simulink model "DC_motor"  (R2021a)
settings: Solver=VariableStepAuto  StartTime=0.0  StopTime=1  RelTol=1e-3
libraries: fl_lib x45, nesl_utility x21, ee_lib x15
settings Model: Creator=vomi  LastModifiedBy=vomi

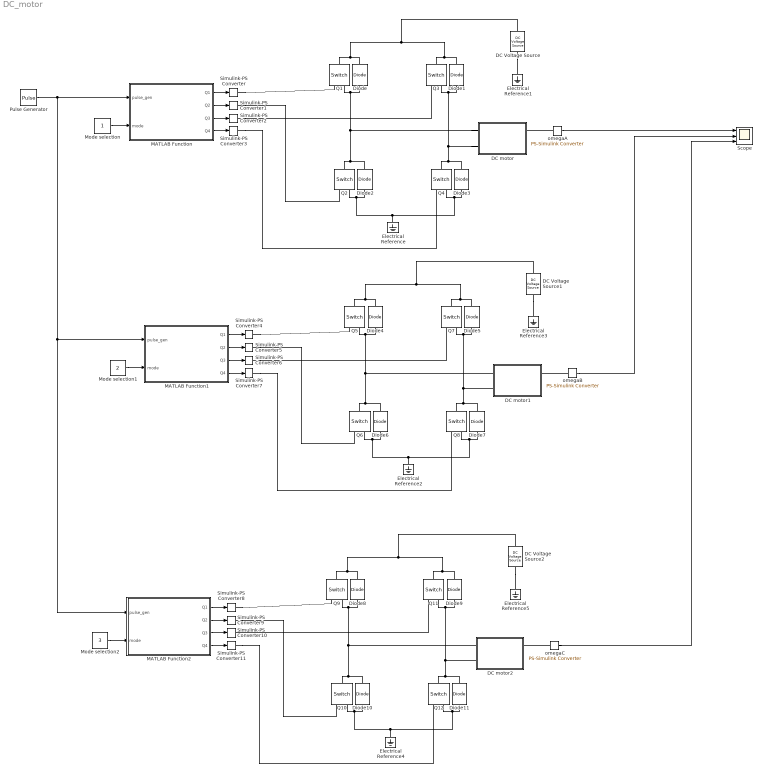
== system DC_motor ==
  DC Voltage Source : ee_lib/Additional Components/SPICE Sources/DC Voltage Source  DC=14.4 V
  DC Voltage Source1 : ee_lib/Additional Components/SPICE Sources/DC Voltage Source  DC=14.4 V
  DC Voltage Source2 : ee_lib/Additional Components/SPICE Sources/DC Voltage Source  DC=14.4 V
  DC motor : Subsystem
  DC motor1 : Subsystem
  DC motor2 : Subsystem
  Diode{,1..11} (12 alike) : ee_lib/Semiconductors & Converters/Diode  ModelType=ee.enum.diode.modelType.pwl  IfMat=[.07, .12, .19, 1.75, 4.24, 7.32, 11.2; .16, .3, .72, 2.14, 4.02, 6.35, 9.12] A  TjVec=[25, 125] degC  VfVec=[.5, .7, .9, 1.3, 1.7, 2.1, 2.5] V  Vf=0.6 V  Ron=0.3 Ohm  Goff=1e-8 S  prmExp=ee.enum.diode.expParam.useTwo  I12=[.0137, .545] A  V12=[.6, .7] V  IS=1e-12 A  ec=1  I1=0.0137 A  V1=0.6 V  RS=0 Ohm  Tmeas=25 degC  N_series=1  N_parallel=1  Rz=0.3 Ohm  BV=inf V  C_param=ee.enum.diode.capParam.fixed  CJ=5 pF  CJ0=5 pF  VJ=1 V  Mgrad=0.5  Vvec=[.1, 10, 100] V  Cvec=[3.5, 1, .4] pF  FC=0.5  Q_param=ee.enum.diode.recoveryParam.off  iRM=-7.15 A  iF=4 A  didt=-750 A/us  trr_factor=3  trr=115 ns  Qrr=150 s*nA  TT=50 ns  tau=100 ns  T_param=ee.enum.diode.temperatureParam.off  IS_T2=1.25e-7 A  I1_T2=0.245 A  V1_T2=0.5 V  Tmeas2=125 degC  EG_param=ee.enum.diode.egapParam.material_si  EG=1.11 eV  XTI_param=ee.enum.diode.xtiParam.pn  XTI=3  dBVdT=0 V/K  enable_faults=ee.enum.faults.faultEnable.no  fault_action=ee.enum.faults.faultAction.none  fault_types=ee.enum.diode.faults.open  tau_fault=1e-3 s  IfMat_faulted=[.07, .12, .19, 1.75, 4.24, 7.32, 11.2; .16, .3, .72, 2.14, 4.02, 6.35, 9.12] A  VfVec_faulted=[.5, .7, .9, 1.3, 1.7, 2.1, 2.5] V  Ropen_faulted=1000 Ohm  Gshort_faulted=1000 1/Ohm  Vf_faulted=0.6 V  Ron_faulted=0.3 Ohm  Goff_faulted=1e-8 S  I12_faulted=[.0137, .545] A  V12_faulted=[.6, .7] V  IS_faulted=1e-12 A  ec_faulted=1  I1_faulted=0.0137 A  V1_faulted=0.6 V  RS_faulted=0 Ohm  Rz_faulted=0.3 Ohm  BV_faulted=inf V  Cscale_faulted=100  enable_temporal_fault=ee.enum.faults.faultEnable.no  t_fault=inf s  enable_behavioral_fault=ee.enum.faults.faultEnable.no  max_permissible_voltage=inf V  n_fail_on_voltage=1  max_permissible_current=inf A  t_fail_on_current=1 s  max_permissible_dVdt=inf V/s  Tdevice=25 degC  i_specify=off  i_priority=None  i=0 A  i_nominal_specify=off  i_nominal_unit=A  i_nominal_value=1  v_specify=off  v_priority=None  v=0 V  v_nominal_specify=off  v_nominal_unit=V  v_nominal_value=1  i_diode_specify=off  i_diode_priority=None  i_diode=0 A  i_diode_nominal_specify=off  i_diode_nominal_unit=A  i_diode_nominal_value=1  v_diode_specify=off  v_diode_priority=None  v_diode=0 V  v_diode_nominal_specify=off  v_diode_nominal_unit=V  v_diode_nominal_value=1  i_capacitor_specify=off  i_capacitor_priority=None  i_capacitor=0 A  i_capacitor_nominal_specify=off  i_capacitor_nominal_unit=A  i_capacitor_nominal_value=1  v_capacitor_specify=off  v_capacitor_priority=None  v_capacitor=0 V  v_capacitor_nominal_specify=off  v_capacitor_nominal_unit=V  v_capacitor_nominal_value=1  power_dissipated_specify=off  power_dissipated_priority=None  power_dissipated=0 W  power_dissipated_nominal_specify=off  power_dissipated_nominal_unit=W  power_dissipated_nominal_value=1  max_permissible_temperature=inf K  t_fail_on_temperature=1 s  thermal_network_parameterization=ee.enum.thermalNetworkTopology.cauer  Rth=[0, 10] K/W  Rth_Foster=[4, 6] K/W  thermal_mass_parameterization=ee.enum.thermalNetwork.timeconstant  thermal_mass=[0, 1] J/K  thermal_mass_Foster=[1.5, 3] J/K  thermal_time_constant=[0, 10] s  thermal_time_constant_Foster=[6, 18] s  thermal_mass_initial_temperatures=[25, 25] degC
  Electrical Reference{,1..5} (6 alike) : fl_lib/Electrical/Electrical Elements/Electrical Reference
  MATLAB Function : MATLAB Function  TreatAsAtomicUnit=on
  MATLAB Function1 : MATLAB Function  TreatAsAtomicUnit=on
  MATLAB Function2 : MATLAB Function  TreatAsAtomicUnit=on
  Mode selection : Constant
  Mode selection1 : Constant  Value=2
  Mode selection2 : Constant  Value=3
  Pulse Generator : DiscretePulseGenerator  PulseType=Time based  Period=1/25.3e3  PulseWidth=30
  Q{1..12} (12 alike) : fl_lib/Electrical/Electrical Elements/Switch  R_closed=0.01 Ohm  G_open=1e-8 1/Ohm  Threshold=0.5  i_specify=off  i_priority=None  i=0 A  i_nominal_specify=off  i_nominal_unit=A  i_nominal_value=1  v_specify=off  v_priority=None  v=0 V  v_nominal_specify=off  v_nominal_unit=V  v_nominal_value=1
  Scope : Scope  NumInputPorts=3
  Simulink-PS Converter{,1..11} (12 alike) : nesl_utility/Simulink-PS Converter  PhysicalDomain=network_engine_domain  SubClassName=ps_input  LeftPortType=input  RightPortType=output  PseudoPeriodic=off  Frequencies=[]  NoiseDistribution=none  NoiseParameters=[]  Unit=1  AffineConversion=off  FilteringAndDerivatives=provide  SimscapeFilterOrder=1  InputFilterTimeConstant=0.001  UdotUserProvided=0
      settings: SourceProductBaseCode=PW,SS
  omegaA : nesl_utility/PS-Simulink Converter  PhysicalDomain=network_engine_domain  SubClassName=ps_output  LeftPortType=input  RightPortType=output  PseudoPeriodic=off  Frequencies=[]  Unit=inherit  AffineConversion=off
      settings: SourceProductBaseCode=PW,SS
  omegaB : nesl_utility/PS-Simulink Converter  PhysicalDomain=network_engine_domain  SubClassName=ps_output  LeftPortType=input  RightPortType=output  PseudoPeriodic=off  Frequencies=[]  Unit=inherit  AffineConversion=off
      settings: SourceProductBaseCode=PW,SS
  omegaC : nesl_utility/PS-Simulink Converter  PhysicalDomain=network_engine_domain  SubClassName=ps_output  LeftPortType=input  RightPortType=output  PseudoPeriodic=off  Frequencies=[]  Unit=inherit  AffineConversion=off
      settings: SourceProductBaseCode=PW,SS
  wires:
  omegaA/1 -> Scope/1
  MATLAB Function/2(Q2) -> Simulink-PS Converter1/1
  MATLAB Function/4(Q4) -> Simulink-PS Converter3/1
  MATLAB Function/3(Q3) -> Simulink-PS Converter2/1
  MATLAB Function/1(Q1) -> Simulink-PS Converter/1
  Mode selection/1 -> MATLAB Function/2(mode)
  MATLAB Function1/4(Q4) -> Simulink-PS Converter7/1
  MATLAB Function1/1(Q1) -> Simulink-PS Converter4/1
  MATLAB Function1/2(Q2) -> Simulink-PS Converter5/1
  Mode selection1/1 -> MATLAB Function1/2(mode)
  MATLAB Function1/3(Q3) -> Simulink-PS Converter6/1
  omegaB/1 -> Scope/2
  Pulse Generator/1 -> MATLAB Function1/1(pulse_gen), MATLAB Function2/1(pulse_gen), MATLAB Function/1(pulse_gen)
  Mode selection2/1 -> MATLAB Function2/2(mode)
  MATLAB Function2/1(Q1) -> Simulink-PS Converter8/1
  MATLAB Function2/4(Q4) -> Simulink-PS Converter11/1
  omegaC/1 -> Scope/3
  MATLAB Function2/3(Q3) -> Simulink-PS Converter10/1
  MATLAB Function2/2(Q2) -> Simulink-PS Converter9/1
  connections:
  omegaA/LConn1 -- DC motor/RConn1
  Diode2/RConn1 -- DC motor/LConn1 -- Diode/LConn1 -- Q1/RConn2 -- Q2/LConn1
  Diode/RConn1 -- Q1/LConn1 -- Q3/LConn1 -- Diode1/RConn1 -- DC Voltage Source/LConn1
  Diode3/RConn1 -- DC motor/LConn2 -- Diode1/LConn1 -- Q3/RConn2 -- Q4/LConn1
  Q2/RConn2 -- Electrical Reference/LConn1 -- Diode3/LConn1 -- Q4/RConn2 -- Diode2/LConn1
  DC Voltage Source/RConn1 -- Electrical Reference1/LConn1
  Simulink-PS Converter/RConn1 -- Q1/RConn1
  Simulink-PS Converter1/RConn1 -- Q2/RConn1
  Simulink-PS Converter2/RConn1 -- Q3/RConn1
  Simulink-PS Converter3/RConn1 -- Q4/RConn1
  DC Voltage Source1/LConn1 -- Q7/LConn1 -- Diode5/RConn1 -- Diode4/RConn1 -- Q5/LConn1
  Q7/RConn2 -- Diode7/RConn1 -- Q8/LConn1 -- DC motor1/LConn2 -- Diode5/LConn1
  Q8/RConn2 -- Diode6/LConn1 -- Q6/RConn2 -- Electrical Reference2/LConn1 -- Diode7/LConn1
  Q5/RConn2 -- Diode6/RConn1 -- Q6/LConn1 -- DC motor1/LConn1 -- Diode4/LConn1
  Simulink-PS Converter6/RConn1 -- Q7/RConn1
  omegaB/LConn1 -- DC motor1/RConn1
  Simulink-PS Converter5/RConn1 -- Q6/RConn1
  DC Voltage Source1/RConn1 -- Electrical Reference3/LConn1
  Simulink-PS Converter4/RConn1 -- Q5/RConn1
  Simulink-PS Converter7/RConn1 -- Q8/RConn1
  Q9/RConn2 -- Diode10/RConn1 -- Q10/LConn1 -- DC motor2/LConn1 -- Diode8/LConn1
  Q12/RConn2 -- Diode11/LConn1 -- Electrical Reference4/LConn1 -- Diode10/LConn1 -- Q10/RConn2
  Q11/RConn2 -- Diode9/LConn1 -- Diode11/RConn1 -- Q12/LConn1 -- DC motor2/LConn2
  Q9/LConn1 -- Diode8/RConn1 -- DC Voltage Source2/LConn1 -- Q11/LConn1 -- Diode9/RConn1
  Simulink-PS Converter9/RConn1 -- Q10/RConn1
  Simulink-PS Converter8/RConn1 -- Q9/RConn1
  Simulink-PS Converter10/RConn1 -- Q11/RConn1
  DC Voltage Source2/RConn1 -- Electrical Reference5/LConn1
  omegaC/LConn1 -- DC motor2/RConn1
  Simulink-PS Converter11/RConn1 -- Q12/RConn1

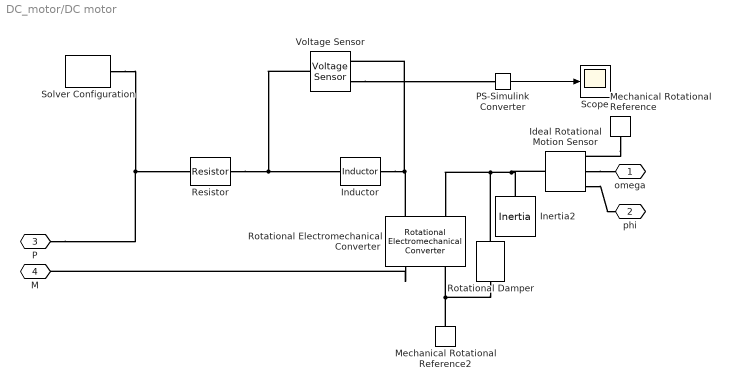
== system DC_motor/DC motor ==
  Ideal Rotational Motion Sensor : fl_lib/Mechanical/Mechanical Sensors/Ideal Rotational Motion Sensor  wrap_angle=simscape.enum.onoff.off  offset=0 rad
  Inductor : fl_lib/Electrical/Electrical Elements/Inductor  l=0.4 mH  r=0 Ohm  g=1e-9 1/Ohm  i_specify=off  i_priority=None  i=0 A  i_nominal_specify=off  i_nominal_unit=A  i_nominal_value=1  v_specify=off  v_priority=None  v=0 V  v_nominal_specify=off  v_nominal_unit=V  v_nominal_value=1  i_L_specify=off  i_L_priority=High  i_L=0 A  i_L_nominal_specify=off  i_L_nominal_unit=A  i_L_nominal_value=1
  Inertia2 : fl_lib/Mechanical/Rotational Elements/Inertia  inertia=71.4e-7 kg*m^2  num_ports=foundation.enum.numPorts2.one  w_specify=off  w_priority=High  w=0 rad/s  w_nominal_specify=off  w_nominal_unit=rad/s  w_nominal_value=1  t_specify=off  t_priority=None  t=0 N*m  t_nominal_specify=off  t_nominal_unit=N*m  t_nominal_value=1
  Mechanical Rotational Reference : fl_lib/Mechanical/Rotational Elements/Mechanical Rotational Reference
  Mechanical Rotational Reference2 : fl_lib/Mechanical/Rotational Elements/Mechanical Rotational Reference
  PS-Simulink Converter : nesl_utility/PS-Simulink Converter  PhysicalDomain=network_engine_domain  SubClassName=ps_output  LeftPortType=input  RightPortType=output  PseudoPeriodic=off  Frequencies=[]  Unit=inherit  AffineConversion=off
      settings: SourceProductBaseCode=PW,SS
  Resistor : fl_lib/Electrical/Electrical Elements/Resistor  R=2.20 Ohm  i_specify=off  i_priority=None  i=0 A  i_nominal_specify=off  i_nominal_unit=A  i_nominal_value=1  v_specify=off  v_priority=None  v=0 V  v_nominal_specify=off  v_nominal_unit=V  v_nominal_value=1
  Rotational Electromechanical Converter : fl_lib/Electrical/Electrical Elements/Rotational Electromechanical Converter  K=5.40e-3 V/rpm  i_specify=off  i_priority=None  i=0 A  i_nominal_specify=off  i_nominal_unit=A  i_nominal_value=1  v_specify=off  v_priority=None  v=0 V  v_nominal_specify=off  v_nominal_unit=V  v_nominal_value=1  t_specify=off  t_priority=None  t=0 N*m  t_nominal_specify=off  t_nominal_unit=N*m  t_nominal_value=1  w_specify=off  w_priority=None  w=0 rad/s  w_nominal_specify=off  w_nominal_unit=rad/s  w_nominal_value=1
  Rotational Damper : fl_lib/Mechanical/Rotational Elements/Rotational Damper  D=0.00002 N*m/(rad/s)  w_specify=off  w_priority=None  w=0 rad/s  w_nominal_specify=off  w_nominal_unit=rad/s  w_nominal_value=1  t_specify=off  t_priority=None  t=0 N*m  t_nominal_specify=off  t_nominal_unit=N*m  t_nominal_value=1
  Scope : Scope
  Solver Configuration : nesl_utility/Solver Configuration  PhysicalDomain=network_engine_domain  SubClassName=solver  LeftPortType=input  RightPortType=generic  Tones=[]  Harmonics=[]  SimulateNoise=off  Profile=off  UseLocalSampling=off  EnableSwitchedLinearOptims=on  FrequencyDomain=off  UseCCode=off  RelTol=0.001  AbsTol=1e-06  MinStep=1e-09  ToWorkspace=off  RevertToSquareIcSolve=off  NumHomotopyIterations=100  PhasorMode=off  PhasorModeNumHarmonics=1  DoDC=off  ResidualTolerance=1e-09  UseLocalSolver=off  LocalSolverChoice=NE_BACKWARD_EULER_ADVANCER  LocalSolverSampleTime=0.001  DoFixedCost=off  MaxNonlinIter=3  MaxModeIter=2  ComputeImpulses=off  ImpulseIterations=2  LinearAlgebra=auto  EquationFormulation=NE_TIME_EF  DelaysMemoryBudget=1024  AutomaticFiltering=on  FilteringTimeConstant=0.001  PartitionStorageMethod=AS_NEEDED  PartitionMemoryBudget=1024  PartitionMethod=ROBUST
      settings: SourceProductBaseCode=PW,SS
  Voltage Sensor : fl_lib/Electrical/Electrical Sensors/Voltage Sensor
  omega : PMIOPort  Side=Right
  phi : PMIOPort  Port=2  Side=Right
  P : PMIOPort  Port=3  Side=Left
  M : PMIOPort  Port=4  Side=Left
  wires:
  PS-Simulink Converter/1 -> Scope/1
  connections:
  Inductor/RConn1 -- Rotational Electromechanical Converter/LConn1 -- Voltage Sensor/RConn2
  Ideal Rotational Motion Sensor/RConn2 -- omega/RConn1
  Resistor/RConn1 -- Voltage Sensor/LConn1 -- Inductor/LConn1
  Inertia2/LConn1 -- Ideal Rotational Motion Sensor/LConn1 -- Rotational Damper/RConn1 -- Rotational Electromechanical Converter/LConn2
  Rotational Electromechanical Converter/RConn1 -- M/RConn1
  Voltage Sensor/RConn1 -- PS-Simulink Converter/LConn1
  Mechanical Rotational Reference/LConn1 -- Ideal Rotational Motion Sensor/RConn1
  Solver Configuration/RConn1 -- P/RConn1 -- Resistor/LConn1
  Mechanical Rotational Reference2/LConn1 -- Rotational Damper/LConn1 -- Rotational Electromechanical Converter/RConn2
  Ideal Rotational Motion Sensor/RConn3 -- phi/RConn1

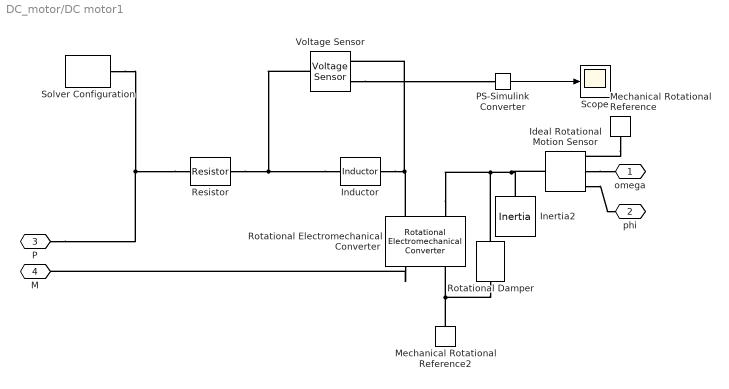
== system DC_motor/DC motor1 ==
  Ideal Rotational Motion Sensor : fl_lib/Mechanical/Mechanical Sensors/Ideal Rotational Motion Sensor  wrap_angle=simscape.enum.onoff.off  offset=0 rad
  Inductor : fl_lib/Electrical/Electrical Elements/Inductor  l=0.4 mH  r=0 Ohm  g=1e-9 1/Ohm  i_specify=off  i_priority=None  i=0 A  i_nominal_specify=off  i_nominal_unit=A  i_nominal_value=1  v_specify=off  v_priority=None  v=0 V  v_nominal_specify=off  v_nominal_unit=V  v_nominal_value=1  i_L_specify=off  i_L_priority=High  i_L=0 A  i_L_nominal_specify=off  i_L_nominal_unit=A  i_L_nominal_value=1
  Inertia2 : fl_lib/Mechanical/Rotational Elements/Inertia  inertia=71.4e-7 kg*m^2  num_ports=foundation.enum.numPorts2.one  w_specify=off  w_priority=High  w=0 rad/s  w_nominal_specify=off  w_nominal_unit=rad/s  w_nominal_value=1  t_specify=off  t_priority=None  t=0 N*m  t_nominal_specify=off  t_nominal_unit=N*m  t_nominal_value=1
  Mechanical Rotational Reference : fl_lib/Mechanical/Rotational Elements/Mechanical Rotational Reference
  Mechanical Rotational Reference2 : fl_lib/Mechanical/Rotational Elements/Mechanical Rotational Reference
  PS-Simulink Converter : nesl_utility/PS-Simulink Converter  PhysicalDomain=network_engine_domain  SubClassName=ps_output  LeftPortType=input  RightPortType=output  PseudoPeriodic=off  Frequencies=[]  Unit=inherit  AffineConversion=off
      settings: SourceProductBaseCode=PW,SS
  Resistor : fl_lib/Electrical/Electrical Elements/Resistor  R=2.20 Ohm  i_specify=off  i_priority=None  i=0 A  i_nominal_specify=off  i_nominal_unit=A  i_nominal_value=1  v_specify=off  v_priority=None  v=0 V  v_nominal_specify=off  v_nominal_unit=V  v_nominal_value=1
  Rotational Electromechanical Converter : fl_lib/Electrical/Electrical Elements/Rotational Electromechanical Converter  K=5.40e-3 V/rpm  i_specify=off  i_priority=None  i=0 A  i_nominal_specify=off  i_nominal_unit=A  i_nominal_value=1  v_specify=off  v_priority=None  v=0 V  v_nominal_specify=off  v_nominal_unit=V  v_nominal_value=1  t_specify=off  t_priority=None  t=0 N*m  t_nominal_specify=off  t_nominal_unit=N*m  t_nominal_value=1  w_specify=off  w_priority=None  w=0 rad/s  w_nominal_specify=off  w_nominal_unit=rad/s  w_nominal_value=1
  Rotational Damper : fl_lib/Mechanical/Rotational Elements/Rotational Damper  D=0.00002 N*m/(rad/s)  w_specify=off  w_priority=None  w=0 rad/s  w_nominal_specify=off  w_nominal_unit=rad/s  w_nominal_value=1  t_specify=off  t_priority=None  t=0 N*m  t_nominal_specify=off  t_nominal_unit=N*m  t_nominal_value=1
  Scope : Scope
  Solver Configuration : nesl_utility/Solver Configuration  PhysicalDomain=network_engine_domain  SubClassName=solver  LeftPortType=input  RightPortType=generic  Tones=[]  Harmonics=[]  SimulateNoise=off  Profile=off  UseLocalSampling=off  EnableSwitchedLinearOptims=on  FrequencyDomain=off  UseCCode=off  RelTol=0.001  AbsTol=1e-06  MinStep=1e-09  ToWorkspace=off  RevertToSquareIcSolve=off  NumHomotopyIterations=100  PhasorMode=off  PhasorModeNumHarmonics=1  DoDC=off  ResidualTolerance=1e-09  UseLocalSolver=off  LocalSolverChoice=NE_BACKWARD_EULER_ADVANCER  LocalSolverSampleTime=0.001  DoFixedCost=off  MaxNonlinIter=3  MaxModeIter=2  ComputeImpulses=off  ImpulseIterations=2  LinearAlgebra=auto  EquationFormulation=NE_TIME_EF  DelaysMemoryBudget=1024  AutomaticFiltering=on  FilteringTimeConstant=0.001  PartitionStorageMethod=AS_NEEDED  PartitionMemoryBudget=1024  PartitionMethod=ROBUST
      settings: SourceProductBaseCode=PW,SS
  Voltage Sensor : fl_lib/Electrical/Electrical Sensors/Voltage Sensor
  omega : PMIOPort  Side=Right
  phi : PMIOPort  Port=2  Side=Right
  P : PMIOPort  Port=3  Side=Left
  M : PMIOPort  Port=4  Side=Left
  wires:
  PS-Simulink Converter/1 -> Scope/1
  connections:
  Inductor/RConn1 -- Voltage Sensor/RConn2 -- Rotational Electromechanical Converter/LConn1
  Ideal Rotational Motion Sensor/RConn2 -- omega/RConn1
  Inductor/LConn1 -- Resistor/RConn1 -- Voltage Sensor/LConn1
  Rotational Electromechanical Converter/LConn2 -- Ideal Rotational Motion Sensor/LConn1 -- Inertia2/LConn1 -- Rotational Damper/RConn1
  Rotational Electromechanical Converter/RConn1 -- M/RConn1
  Voltage Sensor/RConn1 -- PS-Simulink Converter/LConn1
  Mechanical Rotational Reference/LConn1 -- Ideal Rotational Motion Sensor/RConn1
  Resistor/LConn1 -- Solver Configuration/RConn1 -- P/RConn1
  Rotational Electromechanical Converter/RConn2 -- Mechanical Rotational Reference2/LConn1 -- Rotational Damper/LConn1
  Ideal Rotational Motion Sensor/RConn3 -- phi/RConn1

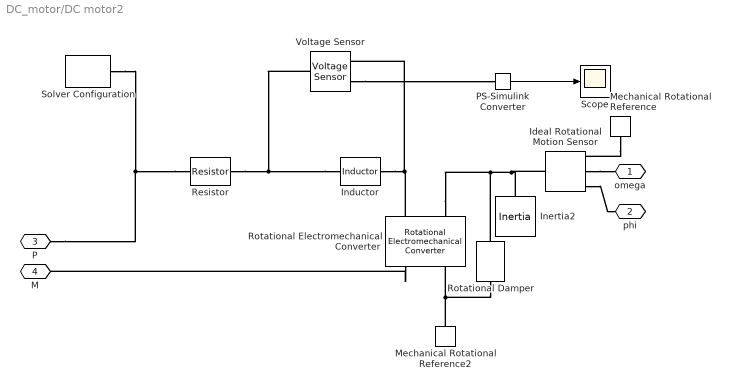
== system DC_motor/DC motor2 ==
  Ideal Rotational Motion Sensor : fl_lib/Mechanical/Mechanical Sensors/Ideal Rotational Motion Sensor  wrap_angle=simscape.enum.onoff.off  offset=0 rad
  Inductor : fl_lib/Electrical/Electrical Elements/Inductor  l=0.4 mH  r=0 Ohm  g=1e-9 1/Ohm  i_specify=off  i_priority=None  i=0 A  i_nominal_specify=off  i_nominal_unit=A  i_nominal_value=1  v_specify=off  v_priority=None  v=0 V  v_nominal_specify=off  v_nominal_unit=V  v_nominal_value=1  i_L_specify=off  i_L_priority=High  i_L=0 A  i_L_nominal_specify=off  i_L_nominal_unit=A  i_L_nominal_value=1
  Inertia2 : fl_lib/Mechanical/Rotational Elements/Inertia  inertia=71.4e-7 kg*m^2  num_ports=foundation.enum.numPorts2.one  w_specify=off  w_priority=High  w=0 rad/s  w_nominal_specify=off  w_nominal_unit=rad/s  w_nominal_value=1  t_specify=off  t_priority=None  t=0 N*m  t_nominal_specify=off  t_nominal_unit=N*m  t_nominal_value=1
  Mechanical Rotational Reference : fl_lib/Mechanical/Rotational Elements/Mechanical Rotational Reference
  Mechanical Rotational Reference2 : fl_lib/Mechanical/Rotational Elements/Mechanical Rotational Reference
  PS-Simulink Converter : nesl_utility/PS-Simulink Converter  PhysicalDomain=network_engine_domain  SubClassName=ps_output  LeftPortType=input  RightPortType=output  PseudoPeriodic=off  Frequencies=[]  Unit=inherit  AffineConversion=off
      settings: SourceProductBaseCode=PW,SS
  Resistor : fl_lib/Electrical/Electrical Elements/Resistor  R=2.20 Ohm  i_specify=off  i_priority=None  i=0 A  i_nominal_specify=off  i_nominal_unit=A  i_nominal_value=1  v_specify=off  v_priority=None  v=0 V  v_nominal_specify=off  v_nominal_unit=V  v_nominal_value=1
  Rotational Electromechanical Converter : fl_lib/Electrical/Electrical Elements/Rotational Electromechanical Converter  K=5.40e-3 V/rpm  i_specify=off  i_priority=None  i=0 A  i_nominal_specify=off  i_nominal_unit=A  i_nominal_value=1  v_specify=off  v_priority=None  v=0 V  v_nominal_specify=off  v_nominal_unit=V  v_nominal_value=1  t_specify=off  t_priority=None  t=0 N*m  t_nominal_specify=off  t_nominal_unit=N*m  t_nominal_value=1  w_specify=off  w_priority=None  w=0 rad/s  w_nominal_specify=off  w_nominal_unit=rad/s  w_nominal_value=1
  Rotational Damper : fl_lib/Mechanical/Rotational Elements/Rotational Damper  D=0.00002 N*m/(rad/s)  w_specify=off  w_priority=None  w=0 rad/s  w_nominal_specify=off  w_nominal_unit=rad/s  w_nominal_value=1  t_specify=off  t_priority=None  t=0 N*m  t_nominal_specify=off  t_nominal_unit=N*m  t_nominal_value=1
  Scope : Scope
  Solver Configuration : nesl_utility/Solver Configuration  PhysicalDomain=network_engine_domain  SubClassName=solver  LeftPortType=input  RightPortType=generic  Tones=[]  Harmonics=[]  SimulateNoise=off  Profile=off  UseLocalSampling=off  EnableSwitchedLinearOptims=on  FrequencyDomain=off  UseCCode=off  RelTol=0.001  AbsTol=1e-06  MinStep=1e-09  ToWorkspace=off  RevertToSquareIcSolve=off  NumHomotopyIterations=100  PhasorMode=off  PhasorModeNumHarmonics=1  DoDC=off  ResidualTolerance=1e-09  UseLocalSolver=off  LocalSolverChoice=NE_BACKWARD_EULER_ADVANCER  LocalSolverSampleTime=0.001  DoFixedCost=off  MaxNonlinIter=3  MaxModeIter=2  ComputeImpulses=off  ImpulseIterations=2  LinearAlgebra=auto  EquationFormulation=NE_TIME_EF  DelaysMemoryBudget=1024  AutomaticFiltering=on  FilteringTimeConstant=0.001  PartitionStorageMethod=AS_NEEDED  PartitionMemoryBudget=1024  PartitionMethod=ROBUST
      settings: SourceProductBaseCode=PW,SS
  Voltage Sensor : fl_lib/Electrical/Electrical Sensors/Voltage Sensor
  omega : PMIOPort  Side=Right
  phi : PMIOPort  Port=2  Side=Right
  P : PMIOPort  Port=3  Side=Left
  M : PMIOPort  Port=4  Side=Left
  wires:
  PS-Simulink Converter/1 -> Scope/1
  connections:
  Inductor/RConn1 -- Voltage Sensor/RConn2 -- Rotational Electromechanical Converter/LConn1
  Ideal Rotational Motion Sensor/RConn2 -- omega/RConn1
  Inductor/LConn1 -- Resistor/RConn1 -- Voltage Sensor/LConn1
  Rotational Electromechanical Converter/LConn2 -- Ideal Rotational Motion Sensor/LConn1 -- Inertia2/LConn1 -- Rotational Damper/RConn1
  Rotational Electromechanical Converter/RConn1 -- M/RConn1
  Voltage Sensor/RConn1 -- PS-Simulink Converter/LConn1
  Mechanical Rotational Reference/LConn1 -- Ideal Rotational Motion Sensor/RConn1
  Resistor/LConn1 -- Solver Configuration/RConn1 -- P/RConn1
  Rotational Electromechanical Converter/RConn2 -- Mechanical Rotational Reference2/LConn1 -- Rotational Damper/LConn1
  Ideal Rotational Motion Sensor/RConn3 -- phi/RConn1

== matlab function DC_motor/MATLAB Function1 ==
  data: pulse_gen input; Q1 output; mode input; Q2 output; Q3 output; Q4 output
function [Q1, Q2, Q3, Q4] = mosfet_drive(pulse_gen, mode)
if pulse_gen == 1 % spínáme
    drive = [1 0 0 1];
else % interval mezi sepnutími, brzdí se
    if mode == 1 % Mode A, Sign-Manitude
        drive = [1 0 1 0];    
    elseif mode == 2 % Mode B, Asynchronous Sign-magnitude
        drive = [1 0 0 0];
    else %Mode C, Lock Anti-Phase
        drive = [0 1 1 0];
    end
end
Q1 = drive(1);
Q2 = drive(2);
Q3 = drive(3);
Q4 = drive(4);
end

== matlab function DC_motor/MATLAB Function ==
  data: pulse_gen input; Q1 output; mode input; Q2 output; Q3 output; Q4 output
function [Q1, Q2, Q3, Q4] = mosfet_drive(pulse_gen, mode)
if pulse_gen == 1 % spínáme
    drive = [1 0 0 1];
else % interval mezi sepnutími, brzdí se
    if mode == 1 % Mode A, Sign-Manitude
        drive = [1 0 1 0];    
    elseif mode == 2 % Mode B, Asynchronous Sign-magnitude
        drive = [1 0 0 0];
    else %Mode C, Lock Anti-Phase
        drive = [0 1 1 0];
    end
end
Q1 = drive(1);
Q2 = drive(2);
Q3 = drive(3);
Q4 = drive(4);
end

== matlab function DC_motor/MATLAB Function2 ==
  data: pulse_gen input; Q1 output; mode input; Q2 output; Q3 output; Q4 output
function [Q1, Q2, Q3, Q4] = mosfet_drive(pulse_gen, mode)
if pulse_gen == 1 % spínáme
    drive = [1 0 0 1];
else % interval mezi sepnutími, brzdí se
    if mode == 1 % Mode A, Sign-Manitude
        drive = [1 0 1 0];    
    elseif mode == 2 % Mode B, Asynchronous Sign-magnitude
        drive = [1 0 0 0];
    else %Mode C, Lock Anti-Phase
        drive = [0 1 1 0];
    end
end
Q1 = drive(1);
Q2 = drive(2);
Q3 = drive(3);
Q4 = drive(4);
end
